simulink model "AODV"  (Simulink 4.00)
settings: Solver=ode45  StartTime=0.0  StopTime=20  RelTol=1e-3
InitFcn:
  | initsim
undefined symbols (not defined in the file or in its folder): WLAN, xPos, yPos
libraries: truetime x8
settings Model: Creator=anton  LastModifiedBy=anton  RTWOptions="-aEnforceIntegerDowncast=1 -aFoldNonRolledExpr=1 -aInlineInvariantSignals=0 -aInlineParameters=0 -aLocalBlockOutputs=1 -aRollThreshold=5 -aGenerateReport=0 -aGenCodeOnly=0 -aRTWVerbose=1 -aIncludeHyperlinkInReport=0 -aLaunchReport=0 -aForceParamTrailComments=0 -aGenerateComments=1 -aIgnoreCustomStorageClasses=1 -aIncHierarchyInIds=0 -aMaxRTWIdLen=31 -aShowEliminatedStatements=0 -aPrefixModelToSubsysFcnNames=1 -aIncDataTypeInIds=0 -aInsertBlockDesc=0 -aSimulinkBlockComments=1 -aInlinedPrmAccess=\"Literals\"  -aSuppressErrorStatus=0 -aModelReferenceCompliant=1 -aSupportNonInlinedSFcns=1 -aSupportContinuousTime=1 -aSupportComplex=1 -aSupportNonFinite=1 -aSupportAbsoluteTime=1 -aTargetPreCompLibLocation=\"\" -aTargetLibSuffix=\"\" -aTargetFcnLib=\"ansi_tfl_tmw.mat\" -aMultiInstanceERTCode=0 -aLogVarNameModifier=\"rt_\" -aERTFirstTimeCompliant=0 -aIsPILTarget=0 -aCombineOutputUpdateFcns=0 -aGenerateASAP2=0 -aGenerateTestInterfaces=0 -aGenerateSampleERTMain=0 -aGenerateFullHeader=1 -aUtilityFuncGeneration=\"Auto\" -aIncludeFileDelimiter=\"Auto\" -aIncludeERTFirstTime=1 -aIncludeMdlTerminateFcn=1 -aPurelyIntegerCode=0 -aERTCustomFileBanners=0 -aRTWCAPIStates=0 -aRTWCAPIParams=0 -aRTWCAPISignals=0 -aMatFileLogging=1 -aGenFloatMathFcnCalls=\"ANSI_C\" -aExtModeMexFile=\"ext_comm\" -aExtModeTransport=0 -aExtModeStaticAllocSize=1000000 -aExtModeTesting=0 -aExtModeStaticAlloc=0 -aExtMode=0"  ExtModeAutoUpdateStatusClock=off  BlockReductionOpt=off

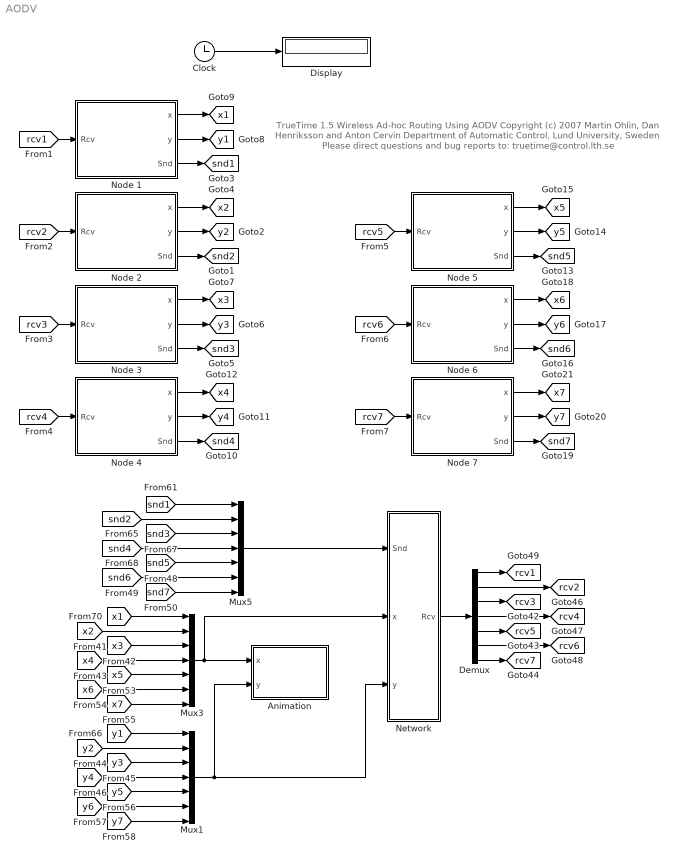
== system AODV ==
  note: TrueTime 1.5  Wireless Ad-hoc Routing Using AODV
      | Copyright (c) 2007
      | Martin Ohlin, Dan Henriksson and Anton Cervin
      | Department of Automatic Control, Lund University, Sweden
      | Please direct questions and bug reports to:  truetime@control.lth.se
  Animation : Subsystem  mask{numMotes=7, xmax=30, ymax=30, ts=0.1, x0=xPos, y0=yPos}
      mask prompts: numMotes "Number of Nodes"; ts "Update period"
      settings: RTWFcnNameOpts=Auto  RTWFileNameOpts=Auto
  Clock : Clock
      settings: DisplayTime=off  Decimation=10
  Demux : Demux  Outputs=7  BusSelectionMode=off
  Display : Display
      settings: Format=short
  Mux1 : Mux  Inputs=7
  Mux3 : Mux  Inputs=7
  Mux5 : Mux  Inputs=7
  Network : Subsystem
      settings: RTWFcnNameOpts=Auto  RTWFileNameOpts=Auto
  Node 1 : Subsystem  mask(MOTE){nodeNbr=1}
      settings: RTWFcnNameOpts=Auto  RTWFileNameOpts=Auto
  Node 2 : Subsystem  mask(MOTE){nodeNbr=2}
      settings: RTWFcnNameOpts=Auto  RTWFileNameOpts=Auto
  Node 3 : Subsystem  mask(MOTE){nodeNbr=3}
      settings: RTWFcnNameOpts=Auto  RTWFileNameOpts=Auto
  Node 4 : Subsystem  mask(MOTE){nodeNbr=4}
      settings: RTWFcnNameOpts=Auto  RTWFileNameOpts=Auto
  Node 5 : Subsystem  mask(MOTE){nodeNbr=5}
      settings: RTWFcnNameOpts=Auto  RTWFileNameOpts=Auto
  Node 6 : Subsystem  mask(MOTE){nodeNbr=6}
      settings: RTWFcnNameOpts=Auto  RTWFileNameOpts=Auto
  Node 7 : Subsystem  mask(MOTE){nodeNbr=7}
      settings: RTWFcnNameOpts=Auto  RTWFileNameOpts=Auto
  tag scope: rcv1=global, rcv2=global, rcv3=global, rcv4=global, rcv5=global, rcv6=global, rcv7=global, snd1=global, snd2=global, snd3=global, snd4=global, snd5=global, snd6=global, snd7=global, x1=global, x2=global, x3=global, x4=global, x5=global, x6=global, x7=global, y1=global, y2=global, y3=global, y4=global, y5=global, y6=global, y7=global
  wires:
  Clock/1 -> Display/1
  Node 1/1(x) -> [x1]
  Node 1/2(y) -> [y1]
  [rcv1] -> Node 1/1(Rcv)
  Node 1/3(Snd) -> [snd1]
  Mux3/1 -> Animation/1(x), Network/2(x)
  [x1] -> Mux3/1
  [x2] -> Mux3/2
  [x3] -> Mux3/3
  [x4] -> Mux3/4
  [x5] -> Mux3/5
  [x6] -> Mux3/6
  [x7] -> Mux3/7
  [y1] -> Mux1/1
  [y2] -> Mux1/2
  [y3] -> Mux1/3
  Mux1/1 -> Animation/2(y), Network/3(y)
  [snd1] -> Mux5/1
  [snd2] -> Mux5/2
  [snd3] -> Mux5/3
  [snd4] -> Mux5/4
  [snd5] -> Mux5/5
  [snd6] -> Mux5/6
  [snd7] -> Mux5/7
  Network/1(Rcv) -> Demux/1
  Mux5/1 -> Network/1(Snd)
  Demux/1 -> [rcv1]
  Demux/3 -> [rcv3]
  Demux/5 -> [rcv5]
  Demux/7 -> [rcv7]
  Demux/2 -> [rcv2]
  Demux/4 -> [rcv4]
  Demux/6 -> [rcv6]
  Node 2/1(x) -> [x2]
  Node 2/2(y) -> [y2]
  [rcv2] -> Node 2/1(Rcv)
  Node 2/3(Snd) -> [snd2]
  Node 3/1(x) -> [x3]
  Node 3/2(y) -> [y3]
  [rcv3] -> Node 3/1(Rcv)
  Node 3/3(Snd) -> [snd3]
  Node 4/1(x) -> [x4]
  Node 4/2(y) -> [y4]
  [rcv4] -> Node 4/1(Rcv)
  Node 4/3(Snd) -> [snd4]
  Node 5/1(x) -> [x5]
  Node 5/2(y) -> [y5]
  [rcv5] -> Node 5/1(Rcv)
  Node 5/3(Snd) -> [snd5]
  Node 6/1(x) -> [x6]
  Node 6/2(y) -> [y6]
  [rcv6] -> Node 6/1(Rcv)
  Node 6/3(Snd) -> [snd6]
  Node 7/1(x) -> [x7]
  Node 7/2(y) -> [y7]
  [rcv7] -> Node 7/1(Rcv)
  Node 7/3(Snd) -> [snd7]
  [y7] -> Mux1/7
  [y6] -> Mux1/6
  [y5] -> Mux1/5
  [y4] -> Mux1/4

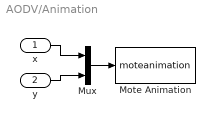
== system AODV/Animation ==
  x : Inport  Port=1  LatchInput=off
  y : Inport  Port=2  LatchInput=off
  Mote Animation : S-Function  FunctionName=moteanimation  Parameters=[numMotes ts xmax ymax] x0 y0  PortCounts=[]  SFunctionModules=''
      settings: DeleteFcn=if ~isempty(findobj('type','figure','name','dblpend1 Animation'));close('dblpend1 Animation'); end;
  Mux : Mux  Inputs=2
  wires:
  Mux/1 -> Mote Animation/1
  y/1 -> Mux/2
  x/1 -> Mux/1

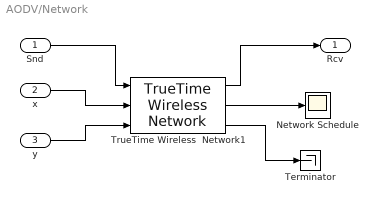
== system AODV/Network ==
  Snd : Inport  Port=1  LatchInput=off
  x : Inport  Port=2  LatchInput=off
  y : Inport  Port=3  LatchInput=off
  Network Schedule : Scope
      settings: TimeRange=0.5  YMin=0.8  YMax=10.7  SaveToWorkspace=off  SaveName=nschedule  MaxDataPoints=5000
  Terminator : Terminator
  TrueTime Wireless  Network1 : truetime/TrueTime Wireless  Network  nwtype=802.11b (WLAN)  nwnbr=1  nnodes=7  rate=1e6  minsize=24  transpower=pow  threshold=thres  pathloss=3.5  use_pathloss_function=off  acktimeout=0.00004  retrylimit=5  error_threshold=codethres
  Rcv : Outport  Port=1
  wires:
  TrueTime Wireless  Network1/1 -> Rcv/1
  Snd/1 -> TrueTime Wireless  Network1/1
  y/1 -> TrueTime Wireless  Network1/3
  x/1 -> TrueTime Wireless  Network1/2
  TrueTime Wireless  Network1/2 -> Network Schedule/1
  TrueTime Wireless  Network1/3 -> Terminator/1

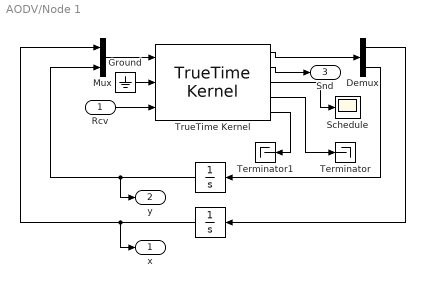
== system AODV/Node 1 ==
  Rcv : Inport  Port=1  LatchInput=off
  " " : Integrator  Orientation=left  ExternalReset=none  InitialConditionSource=internal  InitialCondition=yPos(nodeNbr)  LimitOutput=off  UpperSaturationLimit=inf  LowerSaturationLimit=-inf  ShowSaturationPort=off  ShowStatePort=off  AbsoluteTolerance=auto
  "    " : Integrator  Orientation=left  ExternalReset=none  InitialConditionSource=internal  InitialCondition=xPos(nodeNbr)  LimitOutput=off  UpperSaturationLimit=inf  LowerSaturationLimit=-inf  ShowSaturationPort=off  ShowStatePort=off  AbsoluteTolerance=auto
  Demux : Demux  Outputs=2  BusSelectionMode=off
  Ground : Ground
  Mux : Mux  Inputs=2
  Schedule : Scope
      settings: TickLabels=on  TimeRange=3.5  YMin=1.8  YMax=3.7  SaveToWorkspace=off  SaveName=ScopeData  DataFormat=Array  MaxDataPoints=5000
  Terminator : Terminator
  Terminator1 : Terminator
  TrueTime Kernel : truetime/TrueTime Kernel  sfun=node_init  args=nodeNbr  battery=off  clockdrift=0  clockoffset=0
  x : Outport  Port=1
  y : Outport  Port=2
  Snd : Outport  Port=3
  wires:
  "    "/1 -> x/1, Mux/1
  " "/1 -> y/1, Mux/2
  Demux/1 -> "    "/1
  Demux/2 -> " "/1
  TrueTime Kernel/2 -> Snd/1
  TrueTime Kernel/1 -> Demux/1
  TrueTime Kernel/4 -> Terminator/1
  Mux/1 -> TrueTime Kernel/1
  Rcv/1 -> TrueTime Kernel/3
  Ground/1 -> TrueTime Kernel/2
  TrueTime Kernel/3 -> Schedule/1
  TrueTime Kernel/5 -> Terminator1/1

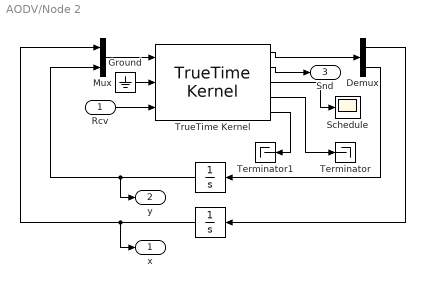
== system AODV/Node 2 ==
  Rcv : Inport  Port=1  LatchInput=off
  " " : Integrator  Orientation=left  ExternalReset=none  InitialConditionSource=internal  InitialCondition=yPos(nodeNbr)  LimitOutput=off  UpperSaturationLimit=inf  LowerSaturationLimit=-inf  ShowSaturationPort=off  ShowStatePort=off  AbsoluteTolerance=auto
  "    " : Integrator  Orientation=left  ExternalReset=none  InitialConditionSource=internal  InitialCondition=xPos(nodeNbr)  LimitOutput=off  UpperSaturationLimit=inf  LowerSaturationLimit=-inf  ShowSaturationPort=off  ShowStatePort=off  AbsoluteTolerance=auto
  Demux : Demux  Outputs=2  BusSelectionMode=off
  Ground : Ground
  Mux : Mux  Inputs=2
  Schedule : Scope
      settings: TickLabels=on  TimeRange=3.5  YMin=1.8  YMax=3.7  SaveToWorkspace=off  SaveName=ScopeData  DataFormat=Array  MaxDataPoints=5000
  Terminator : Terminator
  Terminator1 : Terminator
  TrueTime Kernel : truetime/TrueTime Kernel  sfun=node_init  args=nodeNbr  battery=off  clockdrift=0  clockoffset=0
  x : Outport  Port=1
  y : Outport  Port=2
  Snd : Outport  Port=3
  wires:
  TrueTime Kernel/5 -> Terminator1/1
  TrueTime Kernel/3 -> Schedule/1
  Ground/1 -> TrueTime Kernel/2
  Rcv/1 -> TrueTime Kernel/3
  Mux/1 -> TrueTime Kernel/1
  TrueTime Kernel/4 -> Terminator/1
  TrueTime Kernel/1 -> Demux/1
  TrueTime Kernel/2 -> Snd/1
  Demux/2 -> " "/1
  Demux/1 -> "    "/1
  " "/1 -> Mux/2, y/1
  "    "/1 -> Mux/1, x/1

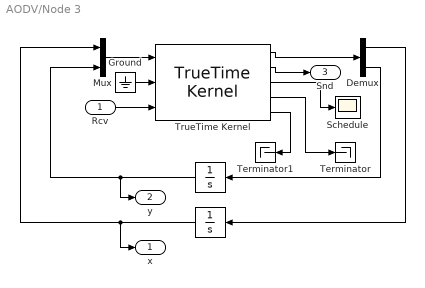
== system AODV/Node 3 ==
  Rcv : Inport  Port=1  LatchInput=off
  " " : Integrator  Orientation=left  ExternalReset=none  InitialConditionSource=internal  InitialCondition=yPos(nodeNbr)  LimitOutput=off  UpperSaturationLimit=inf  LowerSaturationLimit=-inf  ShowSaturationPort=off  ShowStatePort=off  AbsoluteTolerance=auto
  "    " : Integrator  Orientation=left  ExternalReset=none  InitialConditionSource=internal  InitialCondition=xPos(nodeNbr)  LimitOutput=off  UpperSaturationLimit=inf  LowerSaturationLimit=-inf  ShowSaturationPort=off  ShowStatePort=off  AbsoluteTolerance=auto
  Demux : Demux  Outputs=2  BusSelectionMode=off
  Ground : Ground
  Mux : Mux  Inputs=2
  Schedule : Scope
      settings: TickLabels=on  TimeRange=3.5  YMin=1.8  YMax=3.7  SaveToWorkspace=off  SaveName=ScopeData  DataFormat=Array  MaxDataPoints=5000
  Terminator : Terminator
  Terminator1 : Terminator
  TrueTime Kernel : truetime/TrueTime Kernel  sfun=node_init  args=nodeNbr  battery=off  clockdrift=0  clockoffset=0
  x : Outport  Port=1
  y : Outport  Port=2
  Snd : Outport  Port=3
  wires:
  "    "/1 -> x/1, Mux/1
  " "/1 -> y/1, Mux/2
  Demux/1 -> "    "/1
  Demux/2 -> " "/1
  TrueTime Kernel/2 -> Snd/1
  TrueTime Kernel/1 -> Demux/1
  TrueTime Kernel/4 -> Terminator/1
  Mux/1 -> TrueTime Kernel/1
  Rcv/1 -> TrueTime Kernel/3
  Ground/1 -> TrueTime Kernel/2
  TrueTime Kernel/3 -> Schedule/1
  TrueTime Kernel/5 -> Terminator1/1

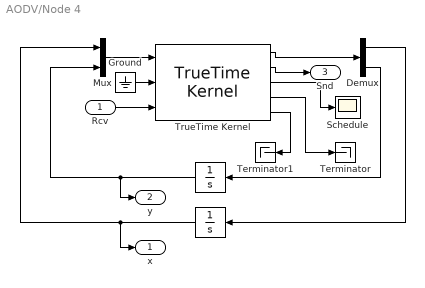
== system AODV/Node 4 ==
  Rcv : Inport  Port=1  LatchInput=off
  " " : Integrator  Orientation=left  ExternalReset=none  InitialConditionSource=internal  InitialCondition=yPos(nodeNbr)  LimitOutput=off  UpperSaturationLimit=inf  LowerSaturationLimit=-inf  ShowSaturationPort=off  ShowStatePort=off  AbsoluteTolerance=auto
  "    " : Integrator  Orientation=left  ExternalReset=none  InitialConditionSource=internal  InitialCondition=xPos(nodeNbr)  LimitOutput=off  UpperSaturationLimit=inf  LowerSaturationLimit=-inf  ShowSaturationPort=off  ShowStatePort=off  AbsoluteTolerance=auto
  Demux : Demux  Outputs=2  BusSelectionMode=off
  Ground : Ground
  Mux : Mux  Inputs=2
  Schedule : Scope
      settings: TickLabels=on  TimeRange=3.5  YMin=1.8  YMax=3.7  SaveToWorkspace=off  SaveName=ScopeData  DataFormat=Array  MaxDataPoints=5000
  Terminator : Terminator
  Terminator1 : Terminator
  TrueTime Kernel : truetime/TrueTime Kernel  sfun=node_init  args=nodeNbr  battery=off  clockdrift=0  clockoffset=0
  x : Outport  Port=1
  y : Outport  Port=2
  Snd : Outport  Port=3
  wires:
  TrueTime Kernel/5 -> Terminator1/1
  TrueTime Kernel/3 -> Schedule/1
  Ground/1 -> TrueTime Kernel/2
  Rcv/1 -> TrueTime Kernel/3
  Mux/1 -> TrueTime Kernel/1
  TrueTime Kernel/4 -> Terminator/1
  TrueTime Kernel/1 -> Demux/1
  TrueTime Kernel/2 -> Snd/1
  Demux/2 -> " "/1
  Demux/1 -> "    "/1
  " "/1 -> Mux/2, y/1
  "    "/1 -> Mux/1, x/1

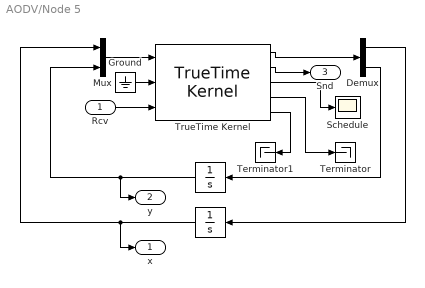
== system AODV/Node 5 ==
  Rcv : Inport  Port=1  LatchInput=off
  " " : Integrator  Orientation=left  ExternalReset=none  InitialConditionSource=internal  InitialCondition=yPos(nodeNbr)  LimitOutput=off  UpperSaturationLimit=inf  LowerSaturationLimit=-inf  ShowSaturationPort=off  ShowStatePort=off  AbsoluteTolerance=auto
  "    " : Integrator  Orientation=left  ExternalReset=none  InitialConditionSource=internal  InitialCondition=xPos(nodeNbr)  LimitOutput=off  UpperSaturationLimit=inf  LowerSaturationLimit=-inf  ShowSaturationPort=off  ShowStatePort=off  AbsoluteTolerance=auto
  Demux : Demux  Outputs=2  BusSelectionMode=off
  Ground : Ground
  Mux : Mux  Inputs=2
  Schedule : Scope
      settings: TickLabels=on  TimeRange=3.5  YMin=1.8  YMax=3.7  SaveToWorkspace=off  SaveName=ScopeData  DataFormat=Array  MaxDataPoints=5000
  Terminator : Terminator
  Terminator1 : Terminator
  TrueTime Kernel : truetime/TrueTime Kernel  sfun=node_init  args=nodeNbr  battery=off  clockdrift=0  clockoffset=0
  x : Outport  Port=1
  y : Outport  Port=2
  Snd : Outport  Port=3
  wires:
  "    "/1 -> x/1, Mux/1
  " "/1 -> y/1, Mux/2
  Demux/1 -> "    "/1
  Demux/2 -> " "/1
  TrueTime Kernel/2 -> Snd/1
  TrueTime Kernel/1 -> Demux/1
  TrueTime Kernel/4 -> Terminator/1
  Mux/1 -> TrueTime Kernel/1
  Rcv/1 -> TrueTime Kernel/3
  Ground/1 -> TrueTime Kernel/2
  TrueTime Kernel/3 -> Schedule/1
  TrueTime Kernel/5 -> Terminator1/1

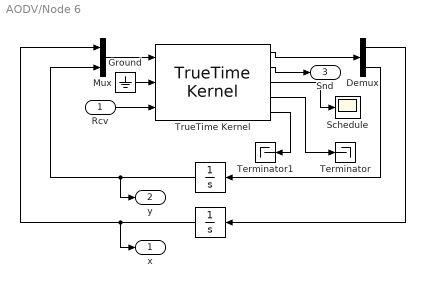
== system AODV/Node 6 ==
  Rcv : Inport  Port=1  LatchInput=off
  " " : Integrator  Orientation=left  ExternalReset=none  InitialConditionSource=internal  InitialCondition=yPos(nodeNbr)  LimitOutput=off  UpperSaturationLimit=inf  LowerSaturationLimit=-inf  ShowSaturationPort=off  ShowStatePort=off  AbsoluteTolerance=auto
  "    " : Integrator  Orientation=left  ExternalReset=none  InitialConditionSource=internal  InitialCondition=xPos(nodeNbr)  LimitOutput=off  UpperSaturationLimit=inf  LowerSaturationLimit=-inf  ShowSaturationPort=off  ShowStatePort=off  AbsoluteTolerance=auto
  Demux : Demux  Outputs=2  BusSelectionMode=off
  Ground : Ground
  Mux : Mux  Inputs=2
  Schedule : Scope
      settings: TickLabels=on  TimeRange=3.5  YMin=1.8  YMax=3.7  SaveToWorkspace=off  SaveName=ScopeData  DataFormat=Array  MaxDataPoints=5000
  Terminator : Terminator
  Terminator1 : Terminator
  TrueTime Kernel : truetime/TrueTime Kernel  sfun=node_init  args=nodeNbr  battery=off  clockdrift=0  clockoffset=0
  x : Outport  Port=1
  y : Outport  Port=2
  Snd : Outport  Port=3
  wires:
  TrueTime Kernel/5 -> Terminator1/1
  TrueTime Kernel/3 -> Schedule/1
  Ground/1 -> TrueTime Kernel/2
  Rcv/1 -> TrueTime Kernel/3
  Mux/1 -> TrueTime Kernel/1
  TrueTime Kernel/4 -> Terminator/1
  TrueTime Kernel/1 -> Demux/1
  TrueTime Kernel/2 -> Snd/1
  Demux/2 -> " "/1
  Demux/1 -> "    "/1
  " "/1 -> Mux/2, y/1
  "    "/1 -> Mux/1, x/1

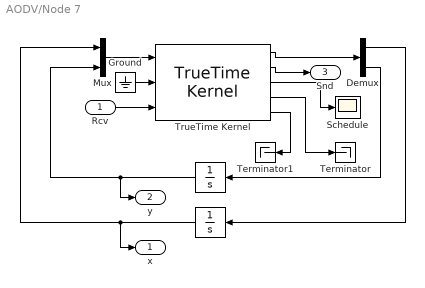
== system AODV/Node 7 ==
  Rcv : Inport  Port=1  LatchInput=off
  " " : Integrator  Orientation=left  ExternalReset=none  InitialConditionSource=internal  InitialCondition=yPos(nodeNbr)  LimitOutput=off  UpperSaturationLimit=inf  LowerSaturationLimit=-inf  ShowSaturationPort=off  ShowStatePort=off  AbsoluteTolerance=auto
  "    " : Integrator  Orientation=left  ExternalReset=none  InitialConditionSource=internal  InitialCondition=xPos(nodeNbr)  LimitOutput=off  UpperSaturationLimit=inf  LowerSaturationLimit=-inf  ShowSaturationPort=off  ShowStatePort=off  AbsoluteTolerance=auto
  Demux : Demux  Outputs=2  BusSelectionMode=off
  Ground : Ground
  Mux : Mux  Inputs=2
  Schedule : Scope
      settings: TickLabels=on  TimeRange=3.5  YMin=1.8  YMax=3.7  SaveToWorkspace=off  SaveName=ScopeData  DataFormat=Array  MaxDataPoints=5000
  Terminator : Terminator
  Terminator1 : Terminator
  TrueTime Kernel : truetime/TrueTime Kernel  sfun=node_init  args=nodeNbr  battery=off  clockdrift=0  clockoffset=0
  x : Outport  Port=1
  y : Outport  Port=2
  Snd : Outport  Port=3
  wires:
  "    "/1 -> x/1, Mux/1
  " "/1 -> y/1, Mux/2
  Demux/1 -> "    "/1
  Demux/2 -> " "/1
  TrueTime Kernel/2 -> Snd/1
  TrueTime Kernel/1 -> Demux/1
  TrueTime Kernel/4 -> Terminator/1
  Mux/1 -> TrueTime Kernel/1
  Rcv/1 -> TrueTime Kernel/3
  Ground/1 -> TrueTime Kernel/2
  TrueTime Kernel/3 -> Schedule/1
  TrueTime Kernel/5 -> Terminator1/1
